simulink model "gm_wlanhdlTimeAndFrequencySynchronization"  (R2025a)
settings: Solver=FixedStepDiscrete  StartTime=0.0  StopTime=stopTime  RelTol=1e-3
InitFcn:
  | wlanFrontEndInit;
undefined symbols (not defined in the file or in its folder): a, b, c, Hd, wlanConfig
libraries: simulink x95, hdlsllib x16, hdlmdlgenlib x12, dspsrcs4 x3, dspsigops x3, dsphdlsigops2 x2, dsphdlfiltering2 x2
(part 4 of 11)

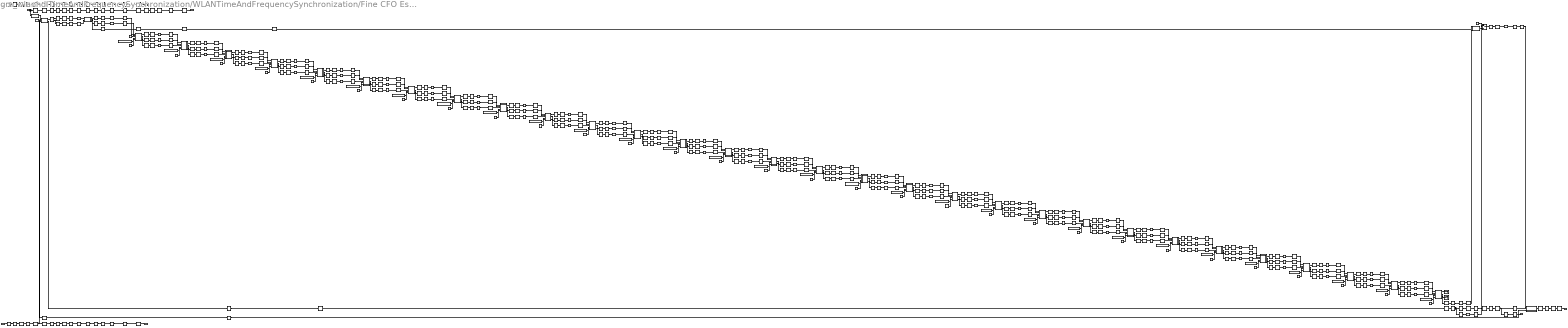
== system gm_wlanhdlTimeAndFrequencySynchronization/WLANTimeAndFrequencySynchronization/Fine CFO Estimation and Correction/Fine CFO Estimation ==
  dataIn : Inport  OutDataTypeStr=fixdt(1, 16, 12)  PortDimensions=1  SampleTime=5e-08
      settings: SignalType=complex
  validIn : Inport  Port=2  OutDataTypeStr=boolean  PortDimensions=1  SampleTime=6.25e-09
  LSTF_start : Inport  Port=3  OutDataTypeStr=boolean  PortDimensions=1  SampleTime=6.25e-09
  rstIn : Inport  Port=4  OutDataTypeStr=boolean  PortDimensions=1  SampleTime=5e-08
  Averager : Subsystem
  Correlator : Subsystem
  Delay10 : Delay  DelayLength=double(64)  InitialCondition=0  SampleTime=5e-08
  Delay{4..5,7,9,13,16..17,21..23,28..31,241,371,391} (17 alike) : RateTransition  InitialCondition=double(0)  OutPortSampleTimeOpt=Multiple of input port sample time  OutPortSampleTimeMultiple=8
  Delay14 : Delay  DelayLength=double(64)  InitialCondition=0  SampleTime=5e-08
  Delay24 : Delay  DelayLength=double(159)  InitialCondition=0  SampleTime=5e-08
  Delay37 : Delay  DelayLength=double(159)  InitialCondition=0  SampleTime=5e-08
  Delay39 : Delay  DelayLength=double(159)  InitialCondition=0  SampleTime=5e-08
  Delay8 : Delay  DelayLength=double(64)  InitialCondition=0  SampleTime=5e-08
  DelayImagInput : RateTransition  InitialCondition=double(0)  OutPortSampleTimeOpt=Multiple of input port sample time  OutPortSampleTimeMultiple=8
  DelayImagInput_absorbed : Delay  DelayLength=0
  DelayQC_Control : RateTransition  InitialCondition=double(0)  OutPortSampleTimeOpt=Multiple of input port sample time  OutPortSampleTimeMultiple=8
  DelayQuadMapper1 : RateTransition  InitialCondition=double(0)  OutPortSampleTimeOpt=Multiple of input port sample time  OutPortSampleTimeMultiple=8
  DelayQuadMapper1_absorbed : Delay  DelayLength=0
  DelayQuadMapper2 : RateTransition  InitialCondition=double(0)  OutPortSampleTimeOpt=Multiple of input port sample time  OutPortSampleTimeMultiple=8
  DelayQuadMapper2_absorbed : Delay  DelayLength=0
  DelayRealInput : RateTransition  InitialCondition=double(0)  OutPortSampleTimeOpt=Multiple of input port sample time  OutPortSampleTimeMultiple=8
  DelayRealInput_absorbed : Delay  DelayLength=0
  DelayValidOut : RateTransition  InitialCondition=double(0)  OutPortSampleTimeOpt=Multiple of input port sample time  OutPortSampleTimeMultiple=8
  Delay_ValidIn : RateTransition  InitialCondition=double(0)  OutPortSampleTimeOpt=Multiple of input port sample time  OutPortSampleTimeMultiple=8
  Initial_ValAng : Constant  Value=0  OutDataTypeStr=fixdt(1, 34, 33)  SampleTime=6.25e-09
  Iteration : Subsystem
  Iteration1 : Subsystem
  Iteration10 : Subsystem
  Iteration11 : Subsystem
  Iteration12 : Subsystem
  Iteration13 : Subsystem
  Iteration14 : Subsystem
  Iteration15 : Subsystem
  Iteration16 : Subsystem
  Iteration17 : Subsystem
  Iteration18 : Subsystem
  Iteration19 : Subsystem
  Iteration2 : Subsystem
  Iteration20 : Subsystem
  Iteration21 : Subsystem
  Iteration22 : Subsystem
  Iteration23 : Subsystem
  Iteration24 : Subsystem
  Iteration25 : Subsystem
  Iteration26 : Subsystem
  Iteration27 : Subsystem
  Iteration28 : Subsystem
  Iteration29 : Subsystem
  Iteration3 : Subsystem
  Iteration4 : Subsystem
  Iteration5 : Subsystem
  Iteration6 : Subsystem
  Iteration7 : Subsystem
  Iteration8 : Subsystem
  Iteration9 : Subsystem
  Iteration_term0 : Terminator
  Iteration_term1 : Terminator
  Output Register : RateTransition  InitialCondition=double(0)  OutPortSampleTimeOpt=Multiple of input port sample time  OutPortSampleTimeMultiple=8
  Output Register_absorbed : Delay  DelayLength=0
  Pipeline{1..32,41..42,51..52,61..62,71..72,81..82,91..92,101..102,110..113,121..122,131..132,141..142,151..152,161..162,171..172,181..182,191..192,201..202,210..213,221..222,231..232,241..242,251..252,261..262,271..272,281..282,291..292} (88 alike) : RateTransition  InitialCondition=double(0)  OutPortSampleTimeOpt=Multiple of input port sample time  OutPortSampleTimeMultiple=8
  Pipeline10_absorbed : Delay  DelayLength=0
  Pipeline10_absorbed1 : Delay  DelayLength=0
  Pipeline10_absorbed2 : Delay  DelayLength=0
  Pipeline11_absorbed : Delay  DelayLength=0
  Pipeline11_absorbed1 : Delay  DelayLength=0
  Pipeline11_absorbed2 : Delay  DelayLength=0
  Pipeline12_absorbed : Delay  DelayLength=0
  Pipeline12_absorbed1 : Delay  DelayLength=0
  Pipeline12_absorbed2 : Delay  DelayLength=0
  Pipeline13_absorbed : Delay  DelayLength=0
  Pipeline13_absorbed1 : Delay  DelayLength=0
  Pipeline13_absorbed2 : Delay  DelayLength=0
  Pipeline14_absorbed : Delay  DelayLength=0
  Pipeline14_absorbed1 : Delay  DelayLength=0
  Pipeline14_absorbed2 : Delay  DelayLength=0
  Pipeline15_absorbed : Delay  DelayLength=0
  Pipeline15_absorbed1 : Delay  DelayLength=0
  Pipeline15_absorbed2 : Delay  DelayLength=0
  Pipeline16_absorbed : Delay  DelayLength=0
  Pipeline16_absorbed1 : Delay  DelayLength=0
  Pipeline16_absorbed2 : Delay  DelayLength=0
  Pipeline17_absorbed : Delay  DelayLength=0
  Pipeline17_absorbed1 : Delay  DelayLength=0
  Pipeline17_absorbed2 : Delay  DelayLength=0
  Pipeline18_absorbed : Delay  DelayLength=0
  Pipeline18_absorbed1 : Delay  DelayLength=0
  Pipeline18_absorbed2 : Delay  DelayLength=0
  Pipeline19_absorbed : Delay  DelayLength=0
  Pipeline19_absorbed1 : Delay  DelayLength=0
  Pipeline19_absorbed2 : Delay  DelayLength=0
  Pipeline1_absorbed : Delay  DelayLength=0
  Pipeline1_absorbed1 : Delay  DelayLength=0
  Pipeline1_absorbed2 : Delay  DelayLength=0
  Pipeline20_absorbed : Delay  DelayLength=0
  Pipeline20_absorbed1 : Delay  DelayLength=0
  Pipeline20_absorbed2 : Delay  DelayLength=0
  Pipeline21_absorbed : Delay  DelayLength=0
  Pipeline21_absorbed1 : Delay  DelayLength=0
  Pipeline21_absorbed2 : Delay  DelayLength=0
  Pipeline22_absorbed : Delay  DelayLength=0
  Pipeline22_absorbed1 : Delay  DelayLength=0
  Pipeline22_absorbed2 : Delay  DelayLength=0
  Pipeline23_absorbed : Delay  DelayLength=0
  Pipeline23_absorbed1 : Delay  DelayLength=0
  Pipeline23_absorbed2 : Delay  DelayLength=0
  Pipeline24_absorbed : Delay  DelayLength=0
  Pipeline24_absorbed1 : Delay  DelayLength=0
  Pipeline24_absorbed2 : Delay  DelayLength=0
  Pipeline25_absorbed : Delay  DelayLength=0
  Pipeline25_absorbed1 : Delay  DelayLength=0
  Pipeline25_absorbed2 : Delay  DelayLength=0
  Pipeline26_absorbed : Delay  DelayLength=0
  Pipeline26_absorbed1 : Delay  DelayLength=0
  Pipeline26_absorbed2 : Delay  DelayLength=0
  Pipeline27_absorbed : Delay  DelayLength=0
  Pipeline27_absorbed1 : Delay  DelayLength=0
  Pipeline27_absorbed2 : Delay  DelayLength=0
  Pipeline28_absorbed : Delay  DelayLength=0
  Pipeline28_absorbed1 : Delay  DelayLength=0
  Pipeline28_absorbed2 : Delay  DelayLength=0
  Pipeline29_absorbed : Delay  DelayLength=0
  Pipeline29_absorbed1 : Delay  DelayLength=0
  Pipeline29_absorbed2 : Delay  DelayLength=0
  Pipeline2_absorbed : Delay  DelayLength=0
  Pipeline2_absorbed1 : Delay  DelayLength=0
  Pipeline2_absorbed2 : Delay  DelayLength=0
  Pipeline30_absorbed : Delay  DelayLength=0
  Pipeline3_absorbed : Delay  DelayLength=0
  Pipeline3_absorbed1 : Delay  DelayLength=0
  Pipeline3_absorbed2 : Delay  DelayLength=0
  Pipeline4_absorbed : Delay  DelayLength=0
  Pipeline4_absorbed1 : Delay  DelayLength=0
  Pipeline4_absorbed2 : Delay  DelayLength=0
  Pipeline5_absorbed : Delay  DelayLength=0
  Pipeline5_absorbed1 : Delay  DelayLength=0
  Pipeline5_absorbed2 : Delay  DelayLength=0
  Pipeline6_absorbed : Delay  DelayLength=0
  Pipeline6_absorbed1 : Delay  DelayLength=0
  Pipeline6_absorbed2 : Delay  DelayLength=0
  Pipeline7_absorbed : Delay  DelayLength=0
  Pipeline7_absorbed1 : Delay  DelayLength=0
  Pipeline7_absorbed2 : Delay  DelayLength=0
  Pipeline8_absorbed : Delay  DelayLength=0
  Pipeline8_absorbed1 : Delay  DelayLength=0
  Pipeline8_absorbed2 : Delay  DelayLength=0
  Pipeline9_absorbed : Delay  DelayLength=0
  Pipeline9_absorbed1 : Delay  DelayLength=0
  Pipeline9_absorbed2 : Delay  DelayLength=0
  QuadrantCorrection : Subsystem
  QuadrantMapper : Subsystem
  Shift Arithmetic : ArithShift  BitShiftNumber=double(7)  BinPtShiftNumber=double(0)
  const : Constant  Value=0.03958342410624027252197265625  OutDataTypeStr=fixdt(0, 31, 33)  SampleTime=6.25e-09
  const1 : Constant  Value=0.0198685242794454097747802734375  OutDataTypeStr=fixdt(0, 31, 33)  SampleTime=6.25e-09
  const10 : Constant  Value=3.88561747968196868896484375e-05  OutDataTypeStr=fixdt(0, 31, 33)  SampleTime=6.25e-09
  const11 : Constant  Value=1.942808739840984344482421875e-05  OutDataTypeStr=fixdt(0, 31, 33)  SampleTime=6.25e-09
  const12 : Constant  Value=9.714043699204921722412109375e-06  OutDataTypeStr=fixdt(0, 31, 33)  SampleTime=6.25e-09
  const13 : Constant  Value=4.85708005726337432861328125e-06  OutDataTypeStr=fixdt(0, 31, 33)  SampleTime=6.25e-09
  const14 : Constant  Value=2.428540028631687164306640625e-06  OutDataTypeStr=fixdt(0, 31, 33)  SampleTime=6.25e-09
  const15 : Constant  Value=1.21421180665493011474609375e-06  OutDataTypeStr=fixdt(0, 31, 33)  SampleTime=6.25e-09
  const16 : Constant  Value=6.07105903327465057373046875e-07  OutDataTypeStr=fixdt(0, 31, 33)  SampleTime=6.25e-09
  const17 : Constant  Value=3.0361115932464599609375e-07  OutDataTypeStr=fixdt(0, 31, 33)  SampleTime=6.25e-09
  const18 : Constant  Value=1.51805579662322998046875e-07  OutDataTypeStr=fixdt(0, 31, 33)  SampleTime=6.25e-09
  const19 : Constant  Value=7.59027898311614990234375e-08  OutDataTypeStr=fixdt(0, 31, 33)  SampleTime=6.25e-09
  const2 : Constant  Value=0.009943947778083384037017822265625  OutDataTypeStr=fixdt(0, 31, 33)  SampleTime=6.25e-09
  const20 : Constant  Value=3.795139491558074951171875e-08  OutDataTypeStr=fixdt(0, 31, 33)  SampleTime=6.25e-09
  const21 : Constant  Value=1.8975697457790374755859375e-08  OutDataTypeStr=fixdt(0, 31, 33)  SampleTime=6.25e-09
  const22 : Constant  Value=9.429641067981719970703125e-09  OutDataTypeStr=fixdt(0, 31, 33)  SampleTime=6.25e-09
  const23 : Constant  Value=4.773028194904327392578125e-09  OutDataTypeStr=fixdt(0, 31, 33)  SampleTime=6.25e-09
  const24 : Constant  Value=2.3283064365386962890625e-09  OutDataTypeStr=fixdt(0, 31, 33)  SampleTime=6.25e-09
  const25 : Constant  Value=1.16415321826934814453125e-09  OutDataTypeStr=fixdt(0, 31, 33)  SampleTime=6.25e-09
  const26 : Constant  Value=5.82076609134674072265625e-10  OutDataTypeStr=fixdt(0, 31, 33)  SampleTime=6.25e-09
  const27 : Constant  Value=3.49245965480804443359375e-10  OutDataTypeStr=fixdt(0, 31, 33)  SampleTime=6.25e-09
  const28 : Constant  Value=0  OutDataTypeStr=fixdt(1, 34, 33)  SampleTime=6.25e-09
  const29 : Constant  Value=0.14758361759595572948455810546875  OutDataTypeStr=fixdt(0, 31, 33)  SampleTime=6.25e-09
  const3 : Constant  Value=0.004973187227733433246612548828125  OutDataTypeStr=fixdt(0, 31, 33)  SampleTime=6.25e-09
  const30 : Constant  Value=0.077979130321182310581207275390625  OutDataTypeStr=fixdt(0, 31, 33)  SampleTime=6.25e-09
  const4 : Constant  Value=0.0024867453612387180328369140625  OutDataTypeStr=fixdt(0, 31, 33)  SampleTime=6.25e-09
  const5 : Constant  Value=0.001243391656316816806793212890625  OutDataTypeStr=fixdt(0, 31, 33)  SampleTime=6.25e-09
  const6 : Constant  Value=0.000621698214672505855560302734375  OutDataTypeStr=fixdt(0, 31, 33)  SampleTime=6.25e-09
  const7 : Constant  Value=0.0003108493983745574951171875  OutDataTypeStr=fixdt(0, 31, 33)  SampleTime=6.25e-09
  const8 : Constant  Value=0.00015542469918727874755859375  OutDataTypeStr=fixdt(0, 31, 33)  SampleTime=6.25e-09
  const9 : Constant  Value=7.7712349593639373779296875e-05  OutDataTypeStr=fixdt(0, 31, 33)  SampleTime=6.25e-09
  cplx2reim : ComplexToRealImag  SampleTime=6.25e-09
  dtc : DataTypeConversion  OutDataTypeStr=fixdt(1, 32, 19)  SampleTime=6.25e-09  SaturateOnIntegerOverflow=off  RndMeth=Floor
  dtc1 : DataTypeConversion  OutDataTypeStr=fixdt(1, 32, 19)  SampleTime=6.25e-09  SaturateOnIntegerOverflow=off  RndMeth=Floor
  in0_repeat{,1..30} (31 alike) : RateTransition  Integrity=off  Deterministic=off  OutPortSampleTimeOpt=Multiple of input port sample time  OutPortSampleTimeMultiple=1/8
  in1_repeat{,1..33} (34 alike) : RateTransition  Integrity=off  Deterministic=off  OutPortSampleTimeOpt=Multiple of input port sample time  OutPortSampleTimeMultiple=1/8
  in2_repeat{,1..31} (32 alike) : RateTransition  Integrity=off  Deterministic=off  OutPortSampleTimeOpt=Multiple of input port sample time  OutPortSampleTimeMultiple=1/8
  in3_repeat{,1..3} (4 alike) : RateTransition  Integrity=off  Deterministic=off  OutPortSampleTimeOpt=Multiple of input port sample time  OutPortSampleTimeMultiple=1/8
  in4_repeat : RateTransition  Integrity=off  Deterministic=off  OutPortSampleTimeOpt=Multiple of input port sample time  OutPortSampleTimeMultiple=1/8
  in4_repeat1 : RateTransition  Integrity=off  Deterministic=off  OutPortSampleTimeOpt=Multiple of input port sample time  OutPortSampleTimeMultiple=1/8
  in4_repeat2 : RateTransition  Integrity=off  Deterministic=off  OutPortSampleTimeOpt=Multiple of input port sample time  OutPortSampleTimeMultiple=1/8
  in5_repeat : RateTransition  Integrity=off  Deterministic=off  OutPortSampleTimeOpt=Multiple of input port sample time  OutPortSampleTimeMultiple=1/8
  in5_repeat1 : RateTransition  Integrity=off  Deterministic=off  OutPortSampleTimeOpt=Multiple of input port sample time  OutPortSampleTimeMultiple=1/8
  in5_repeat2 : RateTransition  Integrity=off  Deterministic=off  OutPortSampleTimeOpt=Multiple of input port sample time  OutPortSampleTimeMultiple=1/8
  in6_repeat : RateTransition  Integrity=off  Deterministic=off  OutPortSampleTimeOpt=Multiple of input port sample time  OutPortSampleTimeMultiple=1/8
  inrepeat : RateTransition  Integrity=off  Deterministic=off  OutPortSampleTimeOpt=Multiple of input port sample time  OutPortSampleTimeMultiple=1/8
  invert_reset : simulink/Logic and Bit Operations/Bitwise Operator  logicop=NOT  UseBitMask=off  BitMask=double(0)  BitMaskRealWorld=Real World Value
  muxAng : Switch  Criteria=u2 ~= 0  Threshold="fi(0,0,1,0,\"hex\",\"0\")"  OutDataTypeStr=fixdt(1, 34, 33)  SampleTime=6.25e-09  SaturateOnIntegerOverflow=off  InputSameDT=off
  rd_{0,2,4..94,97,99..100,102,105,107,113} (100 alike) : Delay  DelayLength=double(1)  InitialCondition=0  SampleTime=6.25e-09
  rd_1 : Delay  DelayLength=double(3)  InitialCondition=0  SampleTime=5e-08
  rd_101 : Delay  DelayLength=double(30)  InitialCondition=0  SampleTime=5e-08
  rd_{95..96,103..104,106,111..112,117..118,121..122} (11 alike) : Delay  DelayLength=double(1)  InitialCondition=0  SampleTime=5e-08
  rd_108 : Delay  DelayLength=double(3)  InitialCondition=0  SampleTime=5e-08
  rd_109 : Delay  DelayLength=double(87)  InitialCondition=0  SampleTime=5e-08
  rd_110 : Delay  DelayLength=double(35)  InitialCondition=0  SampleTime=5e-08
  rd_114 : Delay  DelayLength=double(3)  InitialCondition=0  SampleTime=5e-08
  rd_115 : Delay  DelayLength=double(87)  InitialCondition=0  SampleTime=5e-08
  rd_116 : Delay  DelayLength=double(35)  InitialCondition=0  SampleTime=5e-08
  rd_119 : Delay  DelayLength=double(87)  InitialCondition=0  SampleTime=5e-08
  rd_120 : Delay  DelayLength=double(35)  InitialCondition=0  SampleTime=5e-08
  rd_3 : Delay  DelayLength=double(32)  InitialCondition=0  SampleTime=5e-08
  rd_98 : Delay  DelayLength=double(2)  InitialCondition=0  SampleTime=6.25e-09
  sample FreqOff : Subsystem
  sample FreqOff1 : RateTransition  InitialCondition=double(0)  OutPortSampleTimeOpt=Multiple of input port sample time  OutPortSampleTimeMultiple=8
  sample FreqOff2 : RateTransition  InitialCondition=double(0)  OutPortSampleTimeOpt=Multiple of input port sample time  OutPortSampleTimeMultiple=8
  shift0 : Constant  VectorParams1D=off  OutDataTypeStr=fixdt(0, 6, 0)  SampleTime=6.25e-09
  shift1 : Constant  Value=2  VectorParams1D=off  OutDataTypeStr=fixdt(0, 6, 0)  SampleTime=6.25e-09
  shift10 : Constant  Value=11  VectorParams1D=off  OutDataTypeStr=fixdt(0, 6, 0)  SampleTime=6.25e-09
  shift11 : Constant  Value=12  VectorParams1D=off  OutDataTypeStr=fixdt(0, 6, 0)  SampleTime=6.25e-09
  shift12 : Constant  Value=13  VectorParams1D=off  OutDataTypeStr=fixdt(0, 6, 0)  SampleTime=6.25e-09
  shift13 : Constant  Value=14  VectorParams1D=off  OutDataTypeStr=fixdt(0, 6, 0)  SampleTime=6.25e-09
  shift14 : Constant  Value=15  VectorParams1D=off  OutDataTypeStr=fixdt(0, 6, 0)  SampleTime=6.25e-09
  shift15 : Constant  Value=16  VectorParams1D=off  OutDataTypeStr=fixdt(0, 6, 0)  SampleTime=6.25e-09
  shift16 : Constant  Value=17  VectorParams1D=off  OutDataTypeStr=fixdt(0, 6, 0)  SampleTime=6.25e-09
  shift17 : Constant  Value=18  VectorParams1D=off  OutDataTypeStr=fixdt(0, 6, 0)  SampleTime=6.25e-09
  shift18 : Constant  Value=19  VectorParams1D=off  OutDataTypeStr=fixdt(0, 6, 0)  SampleTime=6.25e-09
  shift19 : Constant  Value=20  VectorParams1D=off  OutDataTypeStr=fixdt(0, 6, 0)  SampleTime=6.25e-09
  shift2 : Constant  Value=3  VectorParams1D=off  OutDataTypeStr=fixdt(0, 6, 0)  SampleTime=6.25e-09
  shift20 : Constant  Value=21  VectorParams1D=off  OutDataTypeStr=fixdt(0, 6, 0)  SampleTime=6.25e-09
  shift21 : Constant  Value=22  VectorParams1D=off  OutDataTypeStr=fixdt(0, 6, 0)  SampleTime=6.25e-09
  shift22 : Constant  Value=23  VectorParams1D=off  OutDataTypeStr=fixdt(0, 6, 0)  SampleTime=6.25e-09
  shift23 : Constant  Value=24  VectorParams1D=off  OutDataTypeStr=fixdt(0, 6, 0)  SampleTime=6.25e-09
  shift24 : Constant  Value=25  VectorParams1D=off  OutDataTypeStr=fixdt(0, 6, 0)  SampleTime=6.25e-09
  shift25 : Constant  Value=26  VectorParams1D=off  OutDataTypeStr=fixdt(0, 6, 0)  SampleTime=6.25e-09
  shift26 : Constant  Value=27  VectorParams1D=off  OutDataTypeStr=fixdt(0, 6, 0)  SampleTime=6.25e-09
  shift27 : Constant  Value=28  VectorParams1D=off  OutDataTypeStr=fixdt(0, 6, 0)  SampleTime=6.25e-09
  shift28 : Constant  Value=29  VectorParams1D=off  OutDataTypeStr=fixdt(0, 6, 0)  SampleTime=6.25e-09
  shift29 : Constant  Value=30  VectorParams1D=off  OutDataTypeStr=fixdt(0, 6, 0)  SampleTime=6.25e-09
  shift3 : Constant  Value=4  VectorParams1D=off  OutDataTypeStr=fixdt(0, 6, 0)  SampleTime=6.25e-09
  shift4 : Constant  Value=5  VectorParams1D=off  OutDataTypeStr=fixdt(0, 6, 0)  SampleTime=6.25e-09
  shift5 : Constant  Value=6  VectorParams1D=off  OutDataTypeStr=fixdt(0, 6, 0)  SampleTime=6.25e-09
  shift6 : Constant  Value=7  VectorParams1D=off  OutDataTypeStr=fixdt(0, 6, 0)  SampleTime=6.25e-09
  shift7 : Constant  Value=8  VectorParams1D=off  OutDataTypeStr=fixdt(0, 6, 0)  SampleTime=6.25e-09
  shift8 : Constant  Value=9  VectorParams1D=off  OutDataTypeStr=fixdt(0, 6, 0)  SampleTime=6.25e-09
  shift9 : Constant  Value=10  VectorParams1D=off  OutDataTypeStr=fixdt(0, 6, 0)  SampleTime=6.25e-09
  zout_corrected_wire : hdlmdlgenlib/Buffer
  Freq : Outport  SampleTime=6.25e-09  VectorParamsAs1DForOutWhenUnconnected=off
  freqValidOut : Outport  Port=2  SampleTime=5e-08  VectorParamsAs1DForOutWhenUnconnected=off
  dataOut : Outport  Port=3  SampleTime=5e-08  VectorParamsAs1DForOutWhenUnconnected=off
  validOut : Outport  Port=4  SampleTime=5e-08  VectorParamsAs1DForOutWhenUnconnected=off
  lstfStart : Outport  Port=5  SampleTime=5e-08  VectorParamsAs1DForOutWhenUnconnected=off
  wires:
  Pipeline22_absorbed1/1 -> in1_repeat20/1
  Pipeline22_absorbed/1 -> in2_repeat20/1
  in1_repeat20/1 -> Iteration20/2(yin)
  rd_57/1 -> Pipeline171/1
  Pipeline13_absorbed1/1 -> in1_repeat11/1
  Pipeline24_absorbed2/1 -> in0_repeat22/1
  Pipeline11_absorbed1/1 -> in1_repeat9/1
  Pipeline26_absorbed1/1 -> in1_repeat24/1
  Pipeline26_absorbed/1 -> in2_repeat24/1
  Pipeline27_absorbed2/1 -> in0_repeat25/1
  Pipeline27_absorbed/1 -> in1_repeat25/1
  rd_71/1 -> Pipeline22/1
  Pipeline28_absorbed/1 -> in2_repeat26/1
  Iteration14/2(yout) -> rd_57/1
  Pipeline29_absorbed1/1 -> in1_repeat27/1
  Iteration8/3(zout) -> rd_40/1
  Pipeline30_absorbed/1 -> in0_repeat28/1
  Pipeline18_absorbed2/1 -> in0_repeat16/1
  Delay37/1 -> Delay10/1
  Iteration25/1(xout) -> rd_89/1
  DelayRealInput_absorbed/1 -> QuadrantMapper/1(xin)
  in1_repeat24/1 -> Iteration24/2(yin)
  Pipeline6/1 -> Pipeline6_absorbed2/1
  rd_78/1 -> Pipeline241/1
  Pipeline1_absorbed/1 -> in6_repeat/1
  Pipeline2_absorbed1/1 -> in1_repeat/1
  in2_repeat/1 -> Iteration/3(zin)
  Iteration17/3(zout) -> rd_67/1
  Pipeline32/1 -> Pipeline3_absorbed1/1
  DelayImagInput_absorbed/1 -> QuadrantMapper/2(yin)
  rd_62/1 -> Pipeline19/1
  in0_repeat3/1 -> Iteration3/1(xin)
  Pipeline281/1 -> Pipeline28_absorbed1/1
  Pipeline62/1 -> Pipeline6_absorbed/1
  in0_repeat4/1 -> Iteration4/1(xin)
  in1_repeat4/1 -> Iteration4/2(yin)
  Pipeline7/1 -> Pipeline7_absorbed2/1
  Pipeline82/1 -> Pipeline8_absorbed/1
  rd_54/1 -> Pipeline161/1
  in2_repeat6/1 -> Iteration6/3(zin)
  Pipeline92/1 -> Pipeline9_absorbed/1
  Pipeline10/1 -> Pipeline10_absorbed2/1
  in0_repeat8/1 -> Iteration8/1(xin)
  in2_repeat15/1 -> Iteration15/3(zin)
  Pipeline111/1 -> Pipeline11_absorbed1/1
  in2_repeat8/1 -> Iteration8/3(zin)
  Pipeline11/1 -> Pipeline11_absorbed2/1
  in0_repeat10/1 -> Iteration10/1(xin)
  Pipeline51/1 -> Pipeline5_absorbed1/1
  Iteration17/2(yout) -> rd_66/1
  Iteration13/2(yout) -> rd_54/1
  Pipeline5_absorbed1/1 -> in1_repeat3/1
  rd_1/1 -> Averager/3(load), in3_repeat/1
  Pipeline12/1 -> Pipeline12_absorbed2/1
  const13/1 -> Iteration13/4(lut_value)
  Pipeline12_absorbed1/1 -> in1_repeat10/1
  rd_100/1 -> DelayQC_Control/1
  Iteration16/2(yout) -> rd_63/1
  Iteration25/3(zout) -> rd_91/1
  in1_repeat17/1 -> Iteration17/2(yin)
  in2_repeat12/1 -> Iteration12/3(zin)
  cplx2reim/1 -> dtc/1
  in0_repeat24/1 -> Iteration24/1(xin)
  Pipeline231/1 -> Pipeline23_absorbed1/1
  rd_10/1 -> Pipeline113/1
  rd_110/1 -> in1_repeat32/1
  Pipeline91/1 -> Pipeline9_absorbed1/1
  Iteration2/1(xout) -> rd_20/1
  rd_12/1 -> Pipeline210/1
  in0_repeat6/1 -> Iteration6/1(xin)
  Iteration25/2(yout) -> rd_90/1
  shift9/1 -> Iteration7/5(idx)
  shift14/1 -> Iteration12/5(idx)
  Pipeline13/1 -> Pipeline13_absorbed2/1
  invert_reset/1 -> rd_98/1
  dtc1/1 -> rd_5/1
  rd_58/1 -> Pipeline172/1
  Iteration1/2(yout) -> rd_18/1
  Pipeline8/1 -> Pipeline8_absorbed2/1
  Pipeline16_absorbed/1 -> in2_repeat14/1
  rd_16/1 -> Pipeline32/1
  in2_repeat19/1 -> Iteration19/3(zin)
  sample FreqOff1/1 -> sample FreqOff/3(rst)
  rd_13/1 -> Pipeline213/1
  Pipeline182/1 -> Pipeline18_absorbed/1
  const20/1 -> Iteration20/4(lut_value)
  Delay14/1 -> rd_108/1
  Pipeline1_absorbed2/1 -> in4_repeat2/1
  rd_9/1 -> Pipeline110/1
  rd_32/1 -> Pipeline9/1
  Pipeline3_absorbed1/1 -> in2_repeat1/1
  const30/1 -> Iteration29/4(lut_value)
  rd_106/1 -> freqValidOut/1
  Iteration29/1(xout) -> rd_11/1
  rd_86/1 -> Pipeline27/1
  Pipeline4_absorbed/1 -> in2_repeat2/1
  in0_repeat/1 -> Iteration/1(xin)
  Pipeline21_absorbed/1 -> in2_repeat19/1
  in3_repeat1/1 -> Delay4/1
  rd_118/1 -> validOut/1
  Iteration8/1(xout) -> rd_38/1
  shift27/1 -> Iteration25/5(idx)
  Pipeline27/1 -> Pipeline27_absorbed2/1
  Shift Arithmetic/1 -> Freq/1
  in0_repeat14/1 -> Iteration14/1(xin)
  in1_repeat15/1 -> Iteration15/2(yin)
  rd_67/1 -> Pipeline202/1
  rd_89/1 -> Pipeline28/1
  Pipeline42/1 -> Pipeline4_absorbed/1
  Pipeline11_absorbed/1 -> in2_repeat9/1
  const15/1 -> Iteration15/4(lut_value)
  const5/1 -> Iteration5/4(lut_value)
  Iteration13/1(xout) -> rd_53/1
  Pipeline1_absorbed1/1 -> in5_repeat2/1
  Iteration27/3(zout) -> rd_99/1
  Pipeline21/1 -> Pipeline21_absorbed2/1
  rd_28/1 -> Pipeline72/1
  Iteration5/1(xout) -> rd_29/1
  Iteration24/3(zout) -> rd_88/1
  rd_102/1 -> Output Register/1
  Initial_ValAng/1 -> muxAng/1
  in4_repeat/1 -> Delay5/1
  rd_81/1 -> Pipeline251/1
  rd_77/1 -> Pipeline24/1
  rd_82/1 -> Pipeline252/1
  rd_75/1 -> Pipeline231/1
  in4_repeat2/1 -> Iteration29/1(xin)
  dtc/1 -> rd_4/1
  rd_0/1 -> Delay241/1
  Iteration9/2(yout) -> rd_42/1
  rd_120/1 -> in3_repeat2/1
  rd_80/1 -> Pipeline25/1
  shift2/1 -> Iteration/5(idx)
  Delay24/1 -> Delay8/1
  rd_29/1 -> Pipeline8/1
  in4_repeat1/1 -> Iteration28/1(xin)
  Pipeline172/1 -> Pipeline17_absorbed/1
  rd_41/1 -> Pipeline12/1
  Pipeline18_absorbed/1 -> in2_repeat16/1
  Iteration9/1(xout) -> rd_41/1
  in0_repeat21/1 -> Iteration21/1(xin)
  Pipeline3/1 -> Pipeline3_absorbed2/1
  Iteration26/3(zout) -> rd_94/1
  Pipeline20_absorbed2/1 -> in0_repeat18/1
  Iteration22/3(zout) -> rd_82/1
  Iteration13/3(zout) -> rd_55/1
  Pipeline9_absorbed1/1 -> in1_repeat7/1
  in3_repeat3/1 -> Delay21/1
  rd_24/1 -> Pipeline61/1
  DelayQuadMapper2/1 -> DelayQuadMapper2_absorbed/1
  Pipeline17_absorbed2/1 -> in0_repeat15/1
  in1_repeat11/1 -> Iteration11/2(yin)
  Pipeline152/1 -> Pipeline15_absorbed/1
  Pipeline292/1 -> Pipeline29_absorbed/1
  QuadrantMapper/1(xout) -> rd_6/1
  Delay241/1 -> Delay24/1
  rd_92/1 -> Pipeline29/1
  validIn/1 -> rd_113/1
  DelayValidOut/1 -> rd_95/1
  Pipeline11_absorbed2/1 -> in0_repeat9/1
  Iteration10/3(zout) -> rd_46/1
  rd_90/1 -> Pipeline281/1
  in1_repeat7/1 -> Iteration7/2(yin)
  rd_122/1 -> lstfStart/1
  Pipeline28_absorbed2/1 -> in0_repeat26/1
  Pipeline3_absorbed/1 -> in1_repeat1/1
  shift5/1 -> Iteration3/5(idx)
  Pipeline213/1 -> Pipeline2_absorbed/1
  rd_65/1 -> Pipeline20/1
  in2_repeat4/1 -> Iteration4/3(zin)
  shift21/1 -> Iteration19/5(idx)
  in2_repeat3/1 -> Iteration3/3(zin)
  Iteration6/3(zout) -> rd_34/1
  in2_repeat7/1 -> Iteration7/3(zin)
  Pipeline20_absorbed1/1 -> in1_repeat18/1
  in5_repeat1/1 -> Iteration28/2(yin)
  Iteration14/1(xout) -> rd_56/1
  shift25/1 -> Iteration23/5(idx)
  const1/1 -> Iteration1/4(lut_value)
  in2_repeat31/1 -> Delay16/1
  in0_repeat28/1 -> QuadrantCorrection/1(zin)
  Pipeline222/1 -> Pipeline22_absorbed/1
  Pipeline18_absorbed1/1 -> in1_repeat16/1
  rd_87/1 -> Pipeline271/1
  rd_63/1 -> Pipeline191/1
  Pipeline7_absorbed1/1 -> in1_repeat5/1
  shift10/1 -> Iteration8/5(idx)
  Pipeline17_absorbed/1 -> in2_repeat15/1
  Pipeline232/1 -> Pipeline23_absorbed/1
  Pipeline24_absorbed1/1 -> in1_repeat22/1
  Pipeline30/1 -> Pipeline30_absorbed/1
  shift17/1 -> Iteration15/5(idx)
  Iteration10/2(yout) -> rd_45/1
  Pipeline17_absorbed1/1 -> in1_repeat15/1
  Pipeline16_absorbed2/1 -> in0_repeat14/1
  Iteration7/1(xout) -> rd_35/1
  Pipeline14_absorbed2/1 -> in0_repeat12/1
  const11/1 -> Iteration11/4(lut_value)
  Pipeline5_absorbed/1 -> in2_repeat3/1
  in2_repeat13/1 -> Iteration13/3(zin)
  rd_74/1 -> Pipeline23/1
  Pipeline14/1 -> Pipeline14_absorbed2/1
  shift11/1 -> Iteration9/5(idx)
  Pipeline12_absorbed/1 -> in2_repeat10/1
  dataIn/1 -> in2_repeat28/1, Correlator/1(dataIn)
  Iteration28/2(yout) -> rd_9/1
  Delay10/1 -> rd_114/1
  rd_45/1 -> Pipeline131/1
  Iteration4/3(zout) -> rd_28/1
  Iteration19/1(xout) -> rd_71/1
  Pipeline15_absorbed2/1 -> in0_repeat13/1
  Pipeline24_absorbed/1 -> in2_repeat22/1
  shift22/1 -> Iteration20/5(idx)
  in0_repeat30/1 -> Delay13/1, sample FreqOff2/1
  Pipeline13_absorbed2/1 -> in0_repeat11/1
  rd_98/1 -> muxAng/2
  Pipeline9_absorbed2/1 -> in0_repeat7/1
  Pipeline19_absorbed1/1 -> in1_repeat17/1
  in2_repeat14/1 -> Iteration14/3(zin)
  Pipeline191/1 -> Pipeline19_absorbed1/1
  Iteration16/1(xout) -> rd_62/1
  DelayQC_Control/1 -> rd_101/1
  Iteration11/1(xout) -> rd_47/1
  Pipeline22/1 -> Pipeline22_absorbed2/1
  Pipeline20_absorbed/1 -> in2_repeat18/1
  rstIn/1 -> in1_repeat29/1, Averager/2(rst)
  Delay29/1 -> rd_111/1
  rd_21/1 -> Pipeline51/1
  Iteration20/1(xout) -> rd_74/1
  rd_27/1 -> Pipeline71/1
  Iteration5/3(zout) -> rd_31/1
  Pipeline19_absorbed2/1 -> in0_repeat17/1
  rd_23/1 -> Pipeline6/1
  Iteration15/2(yout) -> rd_60/1
  Pipeline10_absorbed/1 -> in2_repeat8/1
  Iteration15/3(zout) -> rd_61/1
  Pipeline7_absorbed2/1 -> in0_repeat5/1
  rd_11/1 -> Pipeline2/1
  rd_22/1 -> Pipeline52/1
  Pipeline202/1 -> Pipeline20_absorbed/1
  sample FreqOff/1(freqOffOut) -> rd_104/1
  const24/1 -> Iteration24/4(lut_value)
  in2_repeat27/1 -> Iteration27/3(zin)
  rd_4/1 -> DelayRealInput/1
  Delay391/1 -> Delay39/1
  in2_repeat30/1 -> Delay30/1
  Iteration22/1(xout) -> rd_80/1
  rd_47/1 -> Pipeline14/1
  rd_103/1 -> sample FreqOff/1(freqOffIn)
  const3/1 -> Iteration3/4(lut_value)
  Pipeline21_absorbed1/1 -> in1_repeat19/1
  Pipeline15/1 -> Pipeline15_absorbed2/1
  shift0/1 -> Iteration28/5(idx)
  Delay31/1 -> rd_121/1
  Pipeline101/1 -> Pipeline10_absorbed1/1
  Iteration18/1(xout) -> rd_68/1
  Pipeline10_absorbed1/1 -> in1_repeat8/1
  Iteration10/1(xout) -> rd_44/1
  Pipeline26_absorbed2/1 -> in0_repeat24/1
  Pipeline181/1 -> Pipeline18_absorbed1/1
  const23/1 -> Iteration23/4(lut_value)
  muxAng/1 -> rd_102/1
  rd_42/1 -> Pipeline121/1
  in1_repeat33/1 -> Delay17/1
  const25/1 -> Iteration25/4(lut_value)
  rd_56/1 -> Pipeline17/1
  Pipeline26/1 -> Pipeline26_absorbed2/1
  in1_repeat9/1 -> Iteration9/2(yin)
  Pipeline10_absorbed2/1 -> in0_repeat8/1
  in1_repeat29/1 -> sample FreqOff1/1
  Iteration11/2(yout) -> rd_48/1
  Iteration7/2(yout) -> rd_36/1
  in1_repeat14/1 -> Iteration14/2(yin)
  Iteration19/3(zout) -> rd_73/1
  Pipeline8_absorbed/1 -> in2_repeat6/1
  const10/1 -> Iteration10/4(lut_value)
  Delay7/1 -> rd_109/1
  const12/1 -> Iteration12/4(lut_value)
  Pipeline15_absorbed/1 -> in2_repeat13/1
  Iteration7/3(zout) -> rd_37/1
  Iteration12/1(xout) -> rd_50/1
  Pipeline1/1 -> Pipeline1_absorbed2/1
  Iteration12/2(yout) -> rd_51/1
  Pipeline25_absorbed1/1 -> in1_repeat23/1
  cplx2reim/2 -> dtc1/1
  in0_repeat26/1 -> Iteration26/1(xin)
  in1_repeat18/1 -> Iteration18/2(yin)
  rd_49/1 -> Pipeline142/1
  const16/1 -> Iteration16/4(lut_value)
  rd_8/1 -> Pipeline1/1
  rd_107/1 -> Delay391/1
  Delay9/1 -> rd_115/1
  Pipeline16_absorbed1/1 -> in1_repeat14/1
  const29/1 -> Iteration28/4(lut_value)
  Iteration16/3(zout) -> rd_64/1
  Iteration17/1(xout) -> rd_65/1
  in2_repeat26/1 -> Iteration26/3(zin)
  rd_79/1 -> Pipeline242/1
  Pipeline14_absorbed/1 -> in2_repeat12/1
  Delay30/1 -> rd_117/1
  in0_repeat29/1 -> Delay28/1
  in2_repeat2/1 -> Iteration2/3(zin)
  shift23/1 -> Iteration21/5(idx)
  Iteration26/1(xout) -> rd_92/1
  rd_64/1 -> Pipeline192/1
  rd_15/1 -> Pipeline31/1
  shift24/1 -> Iteration22/5(idx)
  rd_52/1 -> Pipeline152/1
  Iteration23/2(yout) -> rd_84/1
  rd_2/1 -> Delay_ValidIn/1
  Pipeline5_absorbed2/1 -> in0_repeat3/1
  const28/1 -> Iteration28/3(zin)
  const22/1 -> Iteration22/4(lut_value)
  Iteration4/2(yout) -> rd_27/1
  Iteration/3(zout) -> rd_16/1
  Iteration22/2(yout) -> rd_81/1
  rd_36/1 -> Pipeline101/1
  Pipeline3_absorbed2/1 -> in0_repeat1/1
  in0_repeat16/1 -> Iteration16/1(xin)
  Iteration24/1(xout) -> rd_86/1
  Pipeline4_absorbed1/1 -> in1_repeat2/1
  Pipeline5/1 -> Pipeline5_absorbed2/1
  shift15/1 -> Iteration13/5(idx)
  const6/1 -> Iteration6/4(lut_value)
  rd_117/1 -> in2_repeat31/1
  QuadrantMapper/3(QA_Control) -> rd_100/1
  Pipeline262/1 -> Pipeline26_absorbed/1
  Iteration23/3(zout) -> rd_85/1
  const14/1 -> Iteration14/4(lut_value)
  in2_repeat20/1 -> Iteration20/3(zin)
  in0_repeat5/1 -> Iteration5/1(xin)
  in1_repeat10/1 -> Iteration10/2(yin)
  Averager/2(validOut) -> rd_2/1
  Pipeline12_absorbed2/1 -> in0_repeat10/1
  in0_repeat15/1 -> Iteration15/1(xin)
  Iteration23/1(xout) -> rd_83/1
  const26/1 -> Iteration26/4(lut_value)
  Iteration21/2(yout) -> rd_78/1
  Iteration27/1(xout) -> Iteration_term0/1
  Pipeline2_absorbed/1 -> in2_repeat/1
  Iteration5/2(yout) -> rd_30/1
  rd_109/1 -> in3_repeat1/1
  Pipeline15_absorbed1/1 -> in1_repeat13/1
  shift6/1 -> Iteration4/5(idx)
  Pipeline25/1 -> Pipeline25_absorbed2/1
  Output Register_absorbed/1 -> zout_corrected_wire/1
  rd_46/1 -> Pipeline132/1
  rd_96/1 -> in0_repeat30/1
  in1_repeat1/1 -> Iteration1/2(yin)
  in0_repeat22/1 -> Iteration22/1(xin)
  Pipeline291/1 -> Pipeline29_absorbed1/1
  Pipeline19/1 -> Pipeline19_absorbed2/1
  Pipeline132/1 -> Pipeline13_absorbed/1
  rd_37/1 -> Pipeline102/1
  rd_95/1 -> in0_repeat29/1
  Pipeline162/1 -> Pipeline16_absorbed/1
  rd_121/1 -> in3_repeat3/1
  const8/1 -> Iteration8/4(lut_value)
  in1_repeat/1 -> Iteration/2(yin)
  Pipeline271/1 -> Pipeline27_absorbed/1
  rd_6/1 -> DelayQuadMapper1/1
  Pipeline112/1 -> Pipeline11_absorbed/1
  rd_60/1 -> Pipeline181/1
  Pipeline23_absorbed2/1 -> in0_repeat21/1
  Delay371/1 -> Delay37/1
  Iteration26/2(yout) -> rd_93/1
  rd_93/1 -> Pipeline291/1
  Iteration21/1(xout) -> rd_77/1
  in2_repeat21/1 -> Iteration21/3(zin)
  Pipeline23_absorbed1/1 -> in1_repeat21/1
  const7/1 -> Iteration7/4(lut_value)
  Pipeline81/1 -> Pipeline8_absorbed1/1
  Pipeline8_absorbed1/1 -> in1_repeat6/1
  Iteration20/3(zout) -> rd_76/1
  rd_84/1 -> Pipeline261/1
  Pipeline24/1 -> Pipeline24_absorbed2/1
  Iteration12/3(zout) -> rd_52/1
  rd_112/1 -> dataOut/1
  Pipeline28_absorbed1/1 -> in1_repeat26/1
  Delay8/1 -> rd_1/1
  Pipeline19_absorbed/1 -> in2_repeat17/1
  Iteration29/2(yout) -> rd_12/1
  shift29/1 -> Iteration27/5(idx)
  in1_repeat32/1 -> Delay29/1
  in0_repeat23/1 -> Iteration23/1(xin)
  Pipeline151/1 -> Pipeline15_absorbed1/1
  Iteration6/1(xout) -> rd_32/1
  Pipeline41/1 -> Pipeline4_absorbed1/1
  Iteration20/2(yout) -> rd_75/1
  Pipeline28/1 -> Pipeline28_absorbed2/1
  DelayQuadMapper1/1 -> DelayQuadMapper1_absorbed/1
  in1_repeat19/1 -> Iteration19/2(yin)
  shift7/1 -> Iteration5/5(idx)
  rd_59/1 -> Pipeline18/1
  const17/1 -> Iteration17/4(lut_value)
  Pipeline23/1 -> Pipeline23_absorbed2/1
  rd_105/1 -> Shift Arithmetic/1
  Iteration3/2(yout) -> rd_24/1
  Pipeline27_absorbed1/1 -> in2_repeat25/1
  shift19/1 -> Iteration17/5(idx)
  Pipeline122/1 -> Pipeline12_absorbed/1
  Pipeline9/1 -> Pipeline9_absorbed2/1
  Pipeline2_absorbed2/1 -> in0_repeat/1
  rd_20/1 -> Pipeline5/1
  DelayQuadMapper2_absorbed/1 -> in5_repeat1/1
  rd_51/1 -> Pipeline151/1
  rd_5/1 -> DelayImagInput/1
  Iteration6/2(yout) -> rd_33/1
  Pipeline241/1 -> Pipeline24_absorbed1/1
  in2_repeat22/1 -> Iteration22/3(zin)
  rd_35/1 -> Pipeline10/1
  rd_116/1 -> in2_repeat30/1
  in2_repeat9/1 -> Iteration9/3(zin)
  shift26/1 -> Iteration24/5(idx)
  rd_73/1 -> Pipeline222/1
  LSTF_start/1 -> rd_0/1
  in2_repeat10/1 -> Iteration10/3(zin)
  rd_30/1 -> Pipeline81/1
  rd_72/1 -> Pipeline221/1
  Pipeline9_absorbed/1 -> in2_repeat7/1
  rd_61/1 -> Pipeline182/1
  in1_repeat6/1 -> Iteration6/2(yin)
  Delay17/1 -> rd_112/1
  const19/1 -> Iteration19/4(lut_value)
  Pipeline25_absorbed/1 -> in2_repeat23/1
  DelayRealInput/1 -> DelayRealInput_absorbed/1
  Pipeline31/1 -> Pipeline3_absorbed/1
  inrepeat/1 -> rd_105/1
  rd_119/1 -> in5_repeat/1
  shift16/1 -> Iteration14/5(idx)
  rd_66/1 -> Pipeline201/1
  Iteration9/3(zout) -> rd_43/1
  in1_repeat16/1 -> Iteration16/2(yin)
  Pipeline4_absorbed2/1 -> in0_repeat2/1
  in1_repeat13/1 -> Iteration13/2(yin)
  in1_repeat22/1 -> Iteration22/2(yin)
  Iteration19/2(yout) -> rd_72/1
  rd_55/1 -> Pipeline162/1
  Iteration/1(xout) -> rd_14/1
  Iteration2/2(yout) -> rd_21/1
  rd_76/1 -> Pipeline232/1
  rd_43/1 -> Pipeline122/1
  rd_104/1 -> inrepeat/1
  Iteration29/3(zout) -> rd_13/1
  DelayImagInput/1 -> DelayImagInput_absorbed/1
  Pipeline212/1 -> Pipeline21_absorbed/1
  Iteration14/3(zout) -> rd_58/1
  rd_68/1 -> Pipeline21/1
  rd_108/1 -> in1_repeat30/1
  in0_repeat12/1 -> Iteration12/1(xin)
  Pipeline22_absorbed2/1 -> in0_repeat20/1
  rd_114/1 -> in2_repeat29/1
  rd_53/1 -> Pipeline16/1
  Delay13/1 -> rd_106/1
  rd_50/1 -> Pipeline15/1
  in2_repeat16/1 -> Iteration16/3(zin)
  in2_repeat18/1 -> Iteration18/3(zin)
  in1_repeat30/1 -> Delay7/1
  zout_corrected_wire/1 -> rd_103/1
  rd_48/1 -> Pipeline141/1
  Iteration21/3(zout) -> rd_79/1
  rd_44/1 -> Pipeline13/1
  in1_repeat2/1 -> Iteration2/2(yin)
  Pipeline21_absorbed2/1 -> in0_repeat19/1
  in2_repeat11/1 -> Iteration11/3(zin)
  Pipeline29_absorbed/1 -> in2_repeat27/1
  QuadrantMapper/2(yout) -> rd_7/1
  in1_repeat12/1 -> Iteration12/2(yin)
  in5_repeat2/1 -> Iteration29/2(yin)
  rd_39/1 -> Pipeline111/1
  Pipeline210/1 -> Pipeline2_absorbed1/1
  in1_repeat8/1 -> Iteration8/2(yin)
  Pipeline29_absorbed2/1 -> in0_repeat27/1
  Iteration/2(yout) -> rd_15/1
  in1_repeat25/1 -> Iteration25/2(yin)
  const9/1 -> Iteration9/4(lut_value)
  Pipeline23_absorbed/1 -> in2_repeat21/1
  in1_repeat3/1 -> Iteration3/2(yin)
  Pipeline221/1 -> Pipeline22_absorbed1/1
  Delay_ValidIn/1 -> rd_3/1
  rd_111/1 -> in1_repeat33/1
  rd_40/1 -> Pipeline112/1
  Pipeline131/1 -> Pipeline13_absorbed1/1
  Pipeline14_absorbed1/1 -> in1_repeat12/1
  Iteration28/1(xout) -> rd_8/1
  const18/1 -> Iteration18/4(lut_value)
  in0_repeat2/1 -> Iteration2/1(xin)
  rd_38/1 -> Pipeline11/1
  rd_115/1 -> in4_repeat/1
  Delay5/1 -> rd_116/1
  rd_18/1 -> Pipeline41/1
  rd_94/1 -> Pipeline292/1
  QuadrantCorrection/1(zout) -> muxAng/3
  in2_repeat23/1 -> Iteration23/3(zin)
  in2_repeat28/1 -> rd_107/1
  Output Register/1 -> Output Register_absorbed/1
  rd_7/1 -> DelayQuadMapper2/1
  shift20/1 -> Iteration18/5(idx)
  Pipeline17/1 -> Pipeline17_absorbed2/1
  Iteration3/3(zout) -> rd_25/1
  rd_34/1 -> Pipeline92/1
  Pipeline7_absorbed/1 -> in2_repeat5/1
  Correlator/1(corrOut) -> Averager/1(corrIn)
  rd_31/1 -> Pipeline82/1
  Pipeline102/1 -> Pipeline10_absorbed/1
  Iteration11/3(zout) -> rd_49/1
  Delay39/1 -> Delay14/1
  rd_33/1 -> Pipeline91/1
  rd_83/1 -> Pipeline26/1
  rd_17/1 -> Pipeline4/1
  Iteration18/2(yout) -> rd_69/1
  Pipeline6_absorbed/1 -> in2_repeat4/1
  rd_91/1 -> Pipeline282/1
  rd_25/1 -> Pipeline62/1
  Pipeline72/1 -> Pipeline7_absorbed/1
  Pipeline282/1 -> Pipeline28_absorbed/1
  rd_3/1 -> in1_repeat31/1
  rd_88/1 -> Pipeline272/1
  shift1/1 -> Iteration29/5(idx)
  const21/1 -> Iteration21/4(lut_value)
  in1_repeat5/1 -> Iteration5/2(yin)
  Pipeline8_absorbed2/1 -> in0_repeat6/1
  Iteration4/1(xout) -> rd_26/1
  in1_repeat31/1 -> DelayValidOut/1, rd_97/1
  const4/1 -> Iteration4/4(lut_value)
  Iteration3/1(xout) -> rd_23/1
  in2_repeat29/1 -> Delay9/1
  shift4/1 -> Iteration2/5(idx)
  in1_repeat23/1 -> Iteration23/2(yin)
  Iteration2/3(zout) -> rd_22/1
  in0_repeat9/1 -> Iteration9/1(xin)
  const2/1 -> Iteration2/4(lut_value)
  in5_repeat/1 -> Delay22/1
  shift3/1 -> Iteration1/5(idx)
  Iteration1/1(xout) -> rd_17/1
  Pipeline201/1 -> Pipeline20_absorbed1/1
  rd_99/1 -> Pipeline30/1
  Pipeline113/1 -> Pipeline1_absorbed/1
  Pipeline13_absorbed/1 -> in2_repeat11/1
  in0_repeat27/1 -> Iteration27/1(xin)
  rd_19/1 -> Pipeline42/1
  in6_repeat/1 -> Iteration29/3(zin)
  sample FreqOff2/1 -> sample FreqOff/2(enb)
  in1_repeat21/1 -> Iteration21/2(yin)
  in0_repeat13/1 -> Iteration13/1(xin)
  in1_repeat26/1 -> Iteration26/2(yin)
  Delay21/1 -> rd_122/1
  Delay16/1 -> rd_118/1
  rd_14/1 -> Pipeline3/1
  in3_repeat/1 -> Delay23/1
  in3_repeat2/1 -> Delay31/1
  rd_97/1 -> invert_reset/1
  Iteration1/3(zout) -> rd_19/1
  Delay28/1 -> rd_96/1
  Pipeline6_absorbed2/1 -> in0_repeat4/1
  in0_repeat17/1 -> Iteration17/1(xin)
  Delay23/1 -> rd_119/1
  rd_70/1 -> Pipeline212/1
  rd_69/1 -> Pipeline211/1
  Iteration24/2(yout) -> rd_87/1
  rd_85/1 -> Pipeline262/1
  in2_repeat1/1 -> Iteration1/3(zin)
  Pipeline71/1 -> Pipeline7_absorbed1/1
  Delay4/1 -> rd_110/1
  DelayQuadMapper1_absorbed/1 -> in4_repeat1/1
  Iteration28/3(zout) -> rd_10/1
  Iteration27/2(yout) -> Iteration_term1/1
  in0_repeat7/1 -> Iteration7/1(xin)
  in1_repeat27/1 -> Iteration27/2(yin)
  Iteration15/1(xout) -> rd_59/1
  Pipeline29/1 -> Pipeline29_absorbed2/1
  Pipeline242/1 -> Pipeline24_absorbed/1
  in2_repeat25/1 -> Iteration25/3(zin)
  rd_113/1 -> Delay371/1
  Pipeline272/1 -> Pipeline27_absorbed1/1
  shift28/1 -> Iteration26/5(idx)
  Delay22/1 -> rd_120/1
  in2_repeat24/1 -> Iteration24/3(zin)
  Pipeline261/1 -> Pipeline26_absorbed1/1
  Pipeline121/1 -> Pipeline12_absorbed1/1
  in1_repeat28/1 -> QuadrantCorrection/2(QA_Control)
  shift12/1 -> Iteration10/5(idx)
  Pipeline251/1 -> Pipeline25_absorbed1/1
  Pipeline252/1 -> Pipeline25_absorbed/1
  in0_repeat18/1 -> Iteration18/1(xin)
  Iteration18/3(zout) -> rd_70/1
  shift13/1 -> Iteration11/5(idx)
  Averager/1(avgCorr) -> cplx2reim/1
  const/1 -> Iteration/4(lut_value)
  in0_repeat20/1 -> Iteration20/1(xin)
  Pipeline2/1 -> Pipeline2_absorbed2/1
  rd_26/1 -> Pipeline7/1
  Pipeline61/1 -> Pipeline6_absorbed1/1
  rd_101/1 -> in1_repeat28/1
  in0_repeat25/1 -> Iteration25/1(xin)
  in0_repeat19/1 -> Iteration19/1(xin)
  Pipeline192/1 -> Pipeline19_absorbed/1
  Pipeline211/1 -> Pipeline21_absorbed1/1
  shift8/1 -> Iteration6/5(idx)
  const27/1 -> Iteration27/4(lut_value)
  in2_repeat5/1 -> Iteration5/3(zin)
  Pipeline4/1 -> Pipeline4_absorbed2/1
  in0_repeat11/1 -> Iteration11/1(xin)
  Pipeline20/1 -> Pipeline20_absorbed2/1
  in2_repeat17/1 -> Iteration17/3(zin)
  Pipeline171/1 -> Pipeline17_absorbed1/1
  Pipeline16/1 -> Pipeline16_absorbed2/1
  in0_repeat1/1 -> Iteration1/1(xin)
  Pipeline52/1 -> Pipeline5_absorbed/1
  Pipeline6_absorbed1/1 -> in1_repeat4/1
  Pipeline18/1 -> Pipeline18_absorbed2/1
  Pipeline161/1 -> Pipeline16_absorbed1/1
  Iteration8/2(yout) -> rd_39/1
  Pipeline110/1 -> Pipeline1_absorbed1/1
  Pipeline141/1 -> Pipeline14_absorbed1/1
  Pipeline142/1 -> Pipeline14_absorbed/1
  shift18/1 -> Iteration16/5(idx)
  Pipeline25_absorbed2/1 -> in0_repeat23/1

== system gm_wlanhdlTimeAndFrequencySynchronization/WLANTimeAndFrequencySynchronization/Fine Time Sync/Correlator ==
  dataIn : Inport  OutDataTypeStr=fixdt(1, 16, 12)  PortDimensions=1  SampleTime=5e-08
      settings: SignalType=complex
  validIn : Inport  Port=2  OutDataTypeStr=boolean  PortDimensions=1  SampleTime=5e-08
  startIn : Inport  Port=3  OutDataTypeStr=boolean  PortDimensions=1  SampleTime=5e-08
  rstIn : Inport  Port=4  OutDataTypeStr=boolean  PortDimensions=1  SampleTime=5e-08
  Delay{,13,15..16} (4 alike) : Delay  DelayLength=double(3)  InitialCondition=0  SampleTime=5e-08
  Delay1 : Delay  DelayLength=double(4)  InitialCondition=0  SampleTime=5e-08
  Delay{3,21,41,131,151} (5 alike) : RateTransition  InitialCondition=double(0)  OutPortSampleTimeOpt=Multiple of input port sample time  OutPortSampleTimeMultiple=8
  Delay2 : Delay  DelayLength=double(4)  InitialCondition=0  SampleTime=5e-08
  Delay22_absorbed : Delay  DelayLength=0
  Delay23_absorbed : Delay  DelayLength=0
  Delay{4..7,24..26} (7 alike) : Delay  DelayLength=double(1)  InitialCondition=0  SampleTime=5e-08
  Delay3_absorbed : Delay  DelayLength=0
  MagnitudeSquared : Subsystem
  corrFilter : Subsystem
  crp_out_delay : Delay  DelayLength=double(1)  InitialCondition=0  SampleTime=6.25e-09
  in0_repeat : RateTransition  Integrity=off  Deterministic=off  OutPortSampleTimeOpt=Multiple of input port sample time  OutPortSampleTimeMultiple=1/8
  in1_repeat : RateTransition  Integrity=off  Deterministic=off  OutPortSampleTimeOpt=Multiple of input port sample time  OutPortSampleTimeMultiple=1/8
  in3_repeat : RateTransition  Integrity=off  Deterministic=off  OutPortSampleTimeOpt=Multiple of input port sample time  OutPortSampleTimeMultiple=1/8
  in4_repeat : RateTransition  Integrity=off  Deterministic=off  OutPortSampleTimeOpt=Multiple of input port sample time  OutPortSampleTimeMultiple=1/8
  corrOut : Outport  SampleTime=5e-08
  corrValid : Outport  Port=2  SampleTime=5e-08
  startOut : Outport  Port=3  SampleTime=5e-08
  dataOut : Outport  Port=4  SampleTime=5e-08
  validOut : Outport  Port=5  SampleTime=5e-08
  wires:
  Delay7/1 -> validOut/1
  Delay4/1 -> corrValid/1
  Delay6/1 -> dataOut/1
  Delay21/1 -> Delay2/1
  Delay22_absorbed/1 -> MagnitudeSquared/1(dataIn)
  startIn/1 -> Delay/1
  Delay/1 -> Delay24/1
  Delay16/1 -> Delay7/1
  Delay23_absorbed/1 -> MagnitudeSquared/2(validIn)
  Delay151/1 -> Delay15/1
  corrFilter/1(dataOut) -> Delay22_absorbed/1
  MagnitudeSquared/1(dataOut) -> crp_out_delay/1
  Delay131/1 -> Delay13/1
  in1_repeat/1 -> Delay21/1
  Delay5/1 -> startOut/1
  rstIn/1 -> corrFilter/3(rst)
  corrFilter/2(validOut) -> Delay23_absorbed/1
  dataIn/1 -> Delay1/1, corrFilter/1(dataIn)
  validIn/1 -> in1_repeat/1, corrFilter/2(validIn)
  Delay24/1 -> in4_repeat/1
  in0_repeat/1 -> Delay151/1
  Delay2/1 -> Delay26/1
  crp_out_delay/1 -> Delay3/1
  Delay3_absorbed/1 -> corrOut/1
  Delay3/1 -> Delay3_absorbed/1
  Delay25/1 -> in0_repeat/1
  in4_repeat/1 -> Delay131/1
  MagnitudeSquared/2(validOut) -> in3_repeat/1
  in3_repeat/1 -> Delay41/1
  Delay26/1 -> Delay16/1
  Delay15/1 -> Delay6/1
  Delay1/1 -> Delay25/1
  Delay41/1 -> Delay4/1
  Delay13/1 -> Delay5/1

== system gm_wlanhdlTimeAndFrequencySynchronization/WLANTimeAndFrequencySynchronization/Fine Time Sync/Peak Searcher ==
  corrIn : Inport  OutDataTypeStr=fixdt(1, 32, 15)  PortDimensions=1  SampleTime=5e-08
  corrValid : Inport  Port=2  OutDataTypeStr=boolean  PortDimensions=1  SampleTime=5e-08
  startIn : Inport  Port=3  OutDataTypeStr=boolean  PortDimensions=1  SampleTime=5e-08
  dataIn : Inport  Port=4  OutDataTypeStr=fixdt(1, 16, 12)  PortDimensions=1  SampleTime=5e-08
      settings: SignalType=complex
  validIn : Inport  Port=5  OutDataTypeStr=boolean  PortDimensions=1  SampleTime=5e-08
  rstIn : Inport  Port=6  OutDataTypeStr=boolean  PortDimensions=1  SampleTime=5e-08
  maxPeakSearcher : Subsystem
  peakDetector : Subsystem
  lstfStart : Outport  SampleTime=6.25e-09
  validOut : Outport  Port=2  SampleTime=6.25e-09
  dataOut : Outport  Port=3  SampleTime=5e-08
  wires:
  maxPeakSearcher/3(dataOut) -> peakDetector/3(dataIn)
  peakDetector/1(lstfStart) -> lstfStart/1
  maxPeakSearcher/2(countRst) -> peakDetector/2(counterRst)
  maxPeakSearcher/1(maxPeakValue) -> peakDetector/1(maxPeakVal)
  peakDetector/3(dataOut) -> dataOut/1
  peakDetector/2(validOut) -> validOut/1
  rstIn/1 -> maxPeakSearcher/6(rstIn)
  maxPeakSearcher/4(validOut) -> peakDetector/4(validIn)
  dataIn/1 -> maxPeakSearcher/5(dataIn)
  validIn/1 -> maxPeakSearcher/4(validIn)
  startIn/1 -> maxPeakSearcher/3(startIn)
  corrValid/1 -> maxPeakSearcher/2(corrValid)
  corrIn/1 -> maxPeakSearcher/1(corrIn)

== system gm_wlanhdlTimeAndFrequencySynchronization/WLANTimeAndFrequencySynchronization/Rx Filter/DTConverter ==
  dataIn1 : Inport  OutDataTypeStr=fixdt(1, 16, 12)  PortDimensions=1  SampleTime=5e-08
      settings: SignalType=complex
  dataIn2 : Inport  Port=2  OutDataTypeStr=fixdt(1, 16, 11)  PortDimensions=1  SampleTime=5e-08
      settings: SignalType=complex
  DTConverter : MATLAB Function  TreatAsAtomicUnit=on
  dataOut : Outport  SampleTime=5e-08  VectorParamsAs1DForOutWhenUnconnected=off
  wires:
  DTConverter/1(dataOut) -> dataOut/1
  dataIn2/1 -> DTConverter/2(dataIn2)
  dataIn1/1 -> DTConverter/1(dataIn1)

== system gm_wlanhdlTimeAndFrequencySynchronization/WLANTimeAndFrequencySynchronization/Coarse CFO Estimation and Correction/Coarse CFO Correction/DTConverter ==
  dataIn1 : Inport  OutDataTypeStr=fixdt(1, 16, 12)  PortDimensions=1  SampleTime=5e-08
      settings: SignalType=complex
  dataIn2 : Inport  Port=2  OutDataTypeStr=fixdt(1, 32, 26)  PortDimensions=1  SampleTime=5e-08
      settings: SignalType=complex
  DTConverter : MATLAB Function  TreatAsAtomicUnit=on
  dataOut : Outport  SampleTime=5e-08  VectorParamsAs1DForOutWhenUnconnected=off
  wires:
  DTConverter/1(dataOut) -> dataOut/1
  dataIn2/1 -> DTConverter/2(dataIn2)
  dataIn1/1 -> DTConverter/1(dataIn1)
